simulink model "try_slew"  (R2020b)
settings: Solver=ode15s  StartTime=0.0  StopTime=5000  MaxStep=0.2  RelTol=1e-8  AbsTol=1e-8
values from neighbouring files (symbols this model uses):
  data = struct()    [config.m]    (also in config6U.m; configSlew.m; mainOffNominal.m = dataFix; statisticalAnalysis.m = dataFix)
libraries: libraryMatlab x4
settings Model: Creator=pacif  LastModifiedBy=pacif

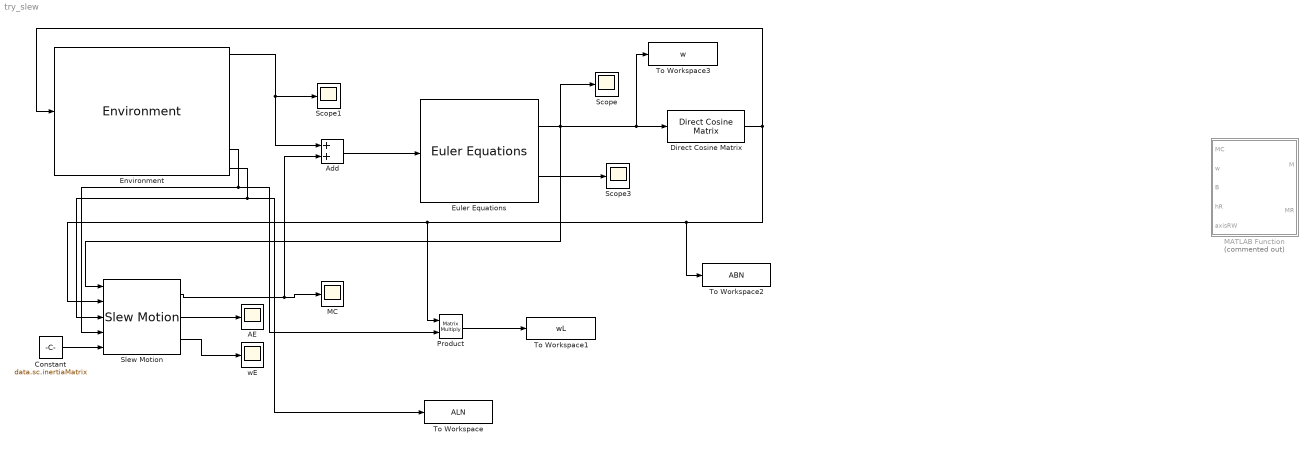
== system try_slew ==
  AE : Scope
  Add : Sum
  Constant : Constant  Value=data.sc.inertiaMatrix
  Direct Cosine Matrix : libraryMatlab/Direct Cosine Matrix  SystemSampleTime=-1  VariantActivationTime=update diagram  Latency=0  AutoFrameSizeCalculation=off
  Environment : libraryMatlab/Environment  SystemSampleTime=-1  VariantActivationTime=update diagram  Latency=0  AutoFrameSizeCalculation=off
  Euler Equations : libraryMatlab/Euler Equations  SystemSampleTime=-1  VariantActivationTime=update diagram  Latency=0  AutoFrameSizeCalculation=off
  MATLAB Function : MATLAB Function  Commented=on  TreatAsAtomicUnit=on
  MC : Scope
  Product : Product  Multiplication=Matrix(*)
  Scope : Scope
  Scope1 : Scope
  Scope3 : Scope
  Slew Motion : libraryMatlab/Slew Motion  SystemSampleTime=-1  VariantActivationTime=update diagram  Latency=0  AutoFrameSizeCalculation=off
      settings: SourceProductBaseCode=SL
  To Workspace : ToWorkspace  VariableName=ALN  SaveFormat=Timeseries  SampleTime=-1
  To Workspace1 : ToWorkspace  VariableName=wL  SaveFormat=Timeseries  SampleTime=-1
  To Workspace2 : ToWorkspace  VariableName=ABN  SaveFormat=Timeseries  SampleTime=-1
  To Workspace3 : ToWorkspace  VariableName=w  SaveFormat=Timeseries  SampleTime=-1
  wE : Scope
  wires:
  Euler Equations/1 -> Slew Motion/1, To Workspace3/1, Direct Cosine Matrix/1, Scope/1
  Direct Cosine Matrix/1 -> To Workspace2/1, Product/1, Slew Motion/2, Environment/1
  Add/1 -> Euler Equations/1
  Environment/1 -> Scope1/1, Add/1
  Euler Equations/2 -> Scope3/1
  Environment/7 -> To Workspace/1, Slew Motion/3
  Environment/6 -> Product/2, Slew Motion/4
  Constant/1 -> Slew Motion/5
  Slew Motion/1 -> MC/1, Add/2
  Slew Motion/2 -> AE/1
  Slew Motion/3 -> wE/1
  Product/1 -> To Workspace1/1

== matlab function try_slew/MATLAB Function ==
  data: MC input; M output; w input; B input; hR input; axisRW input; MR output
function [M,MR] = fun(MC, w, B, hR, axisRW)

MC1 = MC + cross(w,hR*axisRW);

Bx = B(1); By = B(2); Bz = B(3);

% C = [0      Bz      -By     0
%     -Bz     0       Bx      0
%     By      -Bx     0       -1];
% 
% invC = pinv(C);
% 
% u = invC*MC1;
% 
% D = u(1:3)*normB; MR = u(4);
% 
% if abs(D(1)) > 140, D(1) = sign(D(1))*140; end
% if abs(D(2)) > 140, D(2) = sign(D(2))*140; end

Dx = -MC1(2)/Bz; Dy = MC1(1)/Bz;

if abs(Dx) > 140, Dx = sign(Dx)*140; end
if abs(Dy) > 140, Dy = sign(Dy)*140; end

MR = -MC1(3) + By*Dx - Bx*Dy;

if abs(MR) > 18; MR = sign(MR)*18; end
% % if hR >= 0.2 && MR > 0, MR = 0; end
% % if hR <= -0.2 && MR < 0, MR = 0; end

D = [Dx; Dy; 0]; 

M1 = cross(D,B);

M2 = -cross(w,axisRW*hR) - axisRW*MR;


M = M1 + M2;

    


end
